simulink model "TORQUECONTROL"  (R2024b)
settings: configuration reference "STM32H7_Config" (kept outside this file)
settings Model: DataDictionary=Master_Dictionary.sldd  EnableAccessToBaseWorkspace=off  Creator=torni  LastModifiedBy=William
settings ConfigSetRef: SourceName=STM32H7_Config

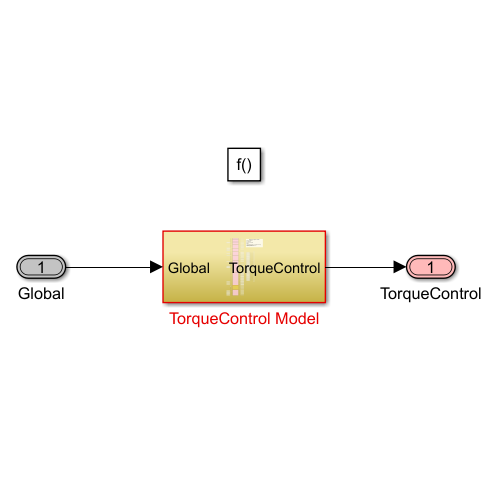
[thumbnail: Simulink's stored preview of the top-level diagram]
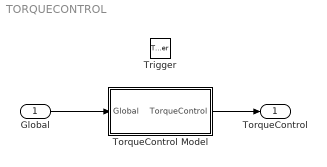
== system TORQUECONTROL ==
  "Global " : Inport  OutDataTypeStr=Bus: Global
  Trigger : TriggerPort  TriggerType=function-call  VariantControl=Variant  PortDimensions=1
  "TorqueControl Model " : Subsystem
  TorqueControl : Outport  OutDataTypeStr=Bus: TorqueControlBus  VectorParamsAs1DForOutWhenUnconnected=off
  wires:
  "Global "/1 -> "TorqueControl Model "/1(Global)
  "TorqueControl Model "/1(TorqueControl) -> TorqueControl/1

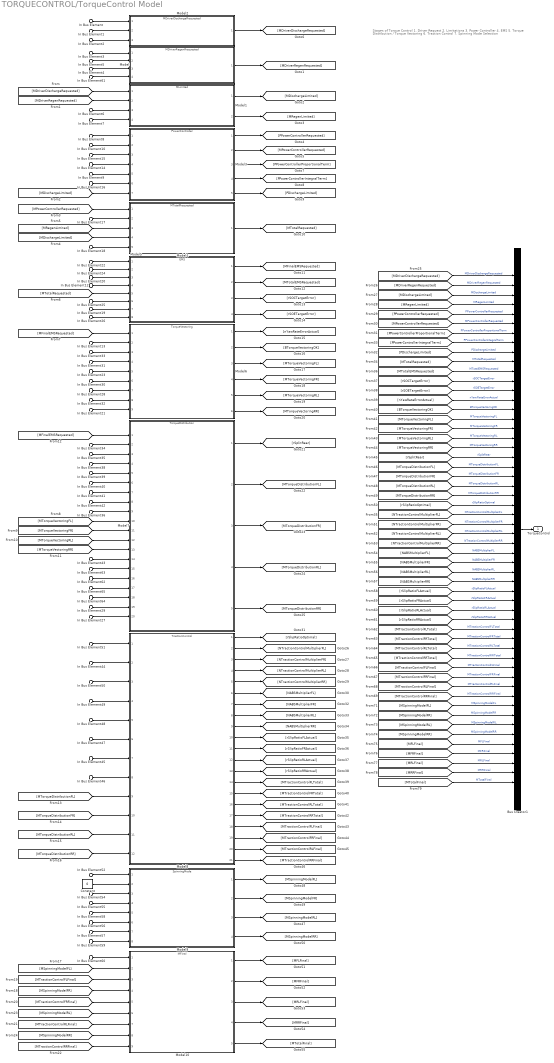
== system TORQUECONTROL/TorqueControl Model  ==
  note: Stages of Torque Control
      | 1. Driver Request
      | 2. Limitations
      | 3. Power Controller
      | 4. EMS
      | 5. Torque Distribution / Torque Vectoring
      | 6. Traction Control
      | 7. Spinning Mode Selection
  In Bus Element{,9,17,28,35,52} (6 alike) : Inport  PortName=Global  Element=SystemsBus.rThrottlePedal
  In Bus Element{1,8,19,23,34,44} (6 alike) : Inport  PortName=Global  Element=SystemsBus.vChassis
  In Bus Element2 : Inport  PortName=Global  Element=SystemsBus.NThrottleMap
  In Bus Element29 : Inport  PortName=Global  Element=SystemsBus.NThrottleMap
  In Bus Element4 : Inport  PortName=Global  Element=SystemsBus.rRegenPaddle
  In Bus Element38 : Inport  PortName=Global  Element=SystemsBus.rRegenPaddle
  In Bus Element5 : Inport  PortName=Global  Element=SystemsBus.PRegen
  In Bus Element10 : Inport  PortName=Global  Element=SystemsBus.NPowerControllerKpSelector
  In Bus Element14 : Inport  PortName=Global  Element=SystemsBus.PActual
  In Bus Element18 : Inport  PortName=Global  Element=SystemsBus.PActual
  In Bus Element16 : Inport  PortName=Global  Element=SystemsBus.PDischarge
  In Bus Element20 : Inport  PortName=Global  Element=SystemsBus.BEMS1000mPoint
  In Bus Element22 : Inport  PortName=Global  Element=SystemsBus.BEMSActivated
  In Bus Element27 : Inport  PortName=Global  Element=SystemsBus.BEMSActivated
  In Bus Element24 : Inport  PortName=Global  Element=SystemsBus.rSOC
  In Bus Element25 : Inport  PortName=Global  Element=SystemsBus.rSOE
  In Bus Element30 : Inport  PortName=Global  Element=SystemsBus.pBrakeMax
  In Bus Element55 : Inport  PortName=Global  Element=SystemsBus.pBrakeMax
  In Bus Element31 : Inport  PortName=Global  Element=SystemsBus.aSteeringAngle
  In Bus Element32 : Inport  PortName=Global  Element=SystemsBus.BTorqueVectoringActivated
  In Bus Element43 : Inport  PortName=Global  Element=SystemsBus.BTorqueVectoringActivated
  In Bus Element33 : Inport  PortName=Global  Element=SystemsBus.rTorqueVectoringMultiplier
  In Bus Element39 : Inport  PortName=Global  Element=SystemsBus.BEncoderErrorRear
  In Bus Element40 : Inport  PortName=Global  Element=SystemsBus.BEncoderErrorFront
  In Bus Element41 : Inport  PortName=Global  Element=SystemsBus.PEngineBraking
  In Bus Element49 : Inport  PortName=Global  Element=SystemsBus.NTractionControlKpSelector
  In Bus Element50 : Inport  PortName=Global  Element=SystemsBus.BTractionControlActivated
  In Bus Element51 : Inport  PortName=Global  Element=SystemsBus.rSteeringAngle
  In Bus Element60 : Inport  PortName=Global  Element=SystemsBus.BSpinningModelActivated
  In Bus Element12 : Inport  PortName=Global  Element=SystemsBus.BEMS995mPoint
  In Bus Element3 : Inport  PortName=Global  Element=BMSSignalsBus.IIVTS
  In Bus Element6 : Inport  PortName=Global  Element=LimitationsBus.rDischargeDerate
  In Bus Element26 : Inport  PortName=Global  Element=LimitationsBus.rDischargeDerate
  In Bus Element7 : Inport  PortName=Global  Element=LimitationsBus.rRegenDerate
  In Bus Element42 : Inport  PortName=Global  Element=LimitationsBus.rRegenDerate
  In Bus Element62 : Inport  PortName=Global  Element=LimitationsBus.rTSTemperatureDerateFR
  In Bus Element63 : Inport  PortName=Global  Element=LimitationsBus.rTSTemperatureDerateFL
  In Bus Element64 : Inport  PortName=Global  Element=LimitationsBus.rTSTemperatureDerateRR
  In Bus Element65 : Inport  PortName=Global  Element=LimitationsBus.rTSTemperatureDerateRL
  In Bus Element15 : Inport  PortName=Global  Element=InverterSignalsBus.InverterRLSignalsBus.VDCInvRL
  In Bus Element36 : Inport  PortName=Global  Element=InverterSignalsBus.InverterRLSignalsBus.VDCInvRL
  In Bus Element61 : Inport  PortName=Global  Element=InverterSignalsBus.InverterRLSignalsBus.VDCInvRL
  In Bus Element58 : Inport  PortName=Global  Element=InverterSignalsBus.InverterRLSignalsBus.nMotorRL
  In Bus Element56 : Inport  PortName=Global  Element=InverterSignalsBus.InverterFLSignalsBus.nMotorFL
  In Bus Element57 : Inport  PortName=Global  Element=InverterSignalsBus.InverterFRSignalsBus.nMotorFR
  In Bus Element59 : Inport  PortName=Global  Element=InverterSignalsBus.InverterRRSignalsBus.nMotorRR
  In Bus Element45 : Inport  PortName=Global  Element=WheelSpeedsBus.vWheelRL
  In Bus Element46 : Inport  PortName=Global  Element=WheelSpeedsBus.vWheelRR
  In Bus Element47 : Inport  PortName=Global  Element=WheelSpeedsBus.vWheelFR
  In Bus Element48 : Inport  PortName=Global  Element=WheelSpeedsBus.vWheelFL
  In Bus Element54 : Inport  PortName=Global  Element=StateflowBus.BReadyToDrive
  In Bus Element13 : Inport  PortName=Global  Element=GPSIMUSignalsBus.gLongitudinalOXTSIMU
  In Bus Element21 : Inport  PortName=Global  Element=GPSIMUSignalsBus.nYawRateOXTSIMU
  Bus Creator1 : BusCreator  Inputs=54  OutDataTypeStr=Bus: TorqueControlBus
  Constant : Constant  Value=0  OutDataTypeStr=boolean
  Model : ModelReference  ModelNameDialog=MDriverRegenRequested.slx  SimulationMode=Normal  ModelReferenceVersion=13.5
  Model1 : ModelReference  ModelNameDialog=MLimited.slx  SimulationMode=Normal  ModelReferenceVersion=13.5
  Model10 : ModelReference  ModelNameDialog=MFinal.slx  SimulationMode=Normal  ModelReferenceVersion=13.5
  Model2 : ModelReference  ModelNameDialog=MDriverDischargeRequested.slx  SimulationMode=Normal  ModelReferenceVersion=13.5
  Model3 : ModelReference  ModelNameDialog=PowerController.slx  SimulationMode=Normal  ModelReferenceVersion=13.5
  Model4 : ModelReference  ModelNameDialog=MTotalRequested.slx  SimulationMode=Normal  ModelReferenceVersion=13.5
  Model5 : ModelReference  ModelNameDialog=EMS.slx  SimulationMode=Normal  ModelReferenceVersion=13.5
  Model6 : ModelReference  ModelNameDialog=TorqueVectoring.slx  SimulationMode=Normal  ModelReferenceVersion=13.5
  Model7 : ModelReference  ModelNameDialog=TorqueDistribution.slx  SimulationMode=Normal  ModelReferenceVersion=13.5
  Model8 : ModelReference  ModelNameDialog=TractionControl.slx  SimulationMode=Normal  ModelReferenceVersion=13.6
  Model9 : ModelReference  ModelNameDialog=SpinningMode.slx  SimulationMode=Normal  ModelReferenceVersion=13.5
  TorqueControl : Outport  OutDataTypeStr=Bus: TorqueControlBus  VectorParamsAs1DForOutWhenUnconnected=off
  wires:
  In Bus Element/1 -> Model2/1
  [MDriverDischargeRequested] -> Model1/1
  Model2/1 -> [MDriverDischargeRequested]
  In Bus Element2/1 -> Model2/3
  In Bus Element1/1 -> Model2/2
  In Bus Element3/1 -> Model/1
  In Bus Element5/1 -> Model/2
  In Bus Element4/1 -> Model/3
  Model/1 -> [MDriverRegenRequested]
  [MDriverRegenRequested] -> Model1/2
  In Bus Element7/1 -> Model1/4
  In Bus Element6/1 -> Model1/3
  Model1/1 -> [MDischargeLimited]
  Model1/2 -> [MRegenLimited]
  Model3/1 -> [PPowerControllerRequested]
  Model3/2 -> [MPowerControllerRequested]
  Model3/3 -> [PPowerControllerProportionalTerm]
  Model3/4 -> [PPowerControllerIntegralTerm]
  Model3/5 -> [PDischargeLimited]
  [MPowerControllerRequested] -> Model4/1
  In Bus Element17/1 -> Model4/2
  In Bus Element18/1 -> Model4/5
  [MDischargeLimited] -> Model4/4
  [MRegenLimited] -> Model4/3
  Model4/1 -> [MTotalRequested]
  In Bus Element12/1 -> Model5/4
  In Bus Element20/1 -> Model5/3
  In Bus Element22/1 -> Model5/1
  [MTotalRequested] -> Model5/5
  In Bus Element25/1 -> Model5/6
  Model5/1 -> [MFinalEMSRequested]
  Model5/2 -> [MTotalEMSRequested]
  Model5/3 -> [rSOCTargetError]
  Model5/4 -> [rSOETargetError]
  In Bus Element13/1 -> Model6/2
  [MFinalEMSRequested] -> Model6/1
  In Bus Element31/1 -> Model6/4
  In Bus Element23/1 -> Model6/5
  In Bus Element30/1 -> Model6/6
  In Bus Element28/1 -> Model6/7
  In Bus Element32/1 -> Model6/8
  In Bus Element21/1 -> Model6/9
  In Bus Element33/1 -> Model6/3
  Model6/1 -> [nYawRateErrorActual]
  Model6/2 -> [BTorqueVectoringOK]
  Model6/3 -> [MTorqueVectoringFL]
  Model6/4 -> [MTorqueVectoringFR]
  Model6/5 -> [MTorqueVectoringRL]
  Model6/6 -> [MTorqueVectoringRR]
  Model7/1 -> [rSplitRear]
  Model7/2 -> [MTorqueDistributionFL]
  Model7/3 -> [MTorqueDistributionFR]
  Model7/4 -> [MTorqueDistributionRL]
  Model7/5 -> [MTorqueDistributionRR]
  Model8/1 -> [rSlipRatioOptimal]
  In Bus Element47/1 -> Model8/6
  In Bus Element56/1 -> Model9/6
  In Bus Element57/1 -> Model9/7
  In Bus Element59/1 -> Model9/8
  In Bus Element58/1 -> Model9/5
  In Bus Element52/1 -> Model9/1
  Constant/1 -> Model9/2
  In Bus Element55/1 -> Model9/4
  Model9/1 -> [MSpinningModelFL]
  Model9/2 -> [MSpinningModelFR]
  Model9/3 -> [MSpinningModelRL]
  Model9/4 -> [MSpinningModelRR]
  Model10/1 -> [MFLFinal]
  Model10/2 -> [MFRFinal]
  Model10/3 -> [MRLFinal]
  Model10/4 -> [MRRFinal]
  [MSpinningModelFL] -> Model10/2
  [MSpinningModelFR] -> Model10/4
  In Bus Element60/1 -> Model10/1
  [MTractionControlFLFinal] -> Model10/3
  [MTractionControlFRFinal] -> Model10/5
  [MTractionControlRLFinal] -> Model10/7
  [MTractionControlRRFinal] -> Model10/9
  [MSpinningModelRL] -> Model10/6
  [MSpinningModelRR] -> Model10/8
  Bus Creator1/1 -> TorqueControl/1
  [MDriverDischargeRequested] -> Bus Creator1/1  "MDriverDischargeRequested"
  [MDriverRegenRequested] -> Bus Creator1/2  "MDriverRegenRequested"
  [MDischargeLimited] -> Bus Creator1/3  "MDischargeLimited"
  [MRegenLimited] -> Bus Creator1/4  "MRegenLimited"
  [PPowerControllerRequested] -> Bus Creator1/5  "PPowerControllerRequested"
  [MPowerControllerRequested] -> Bus Creator1/6  "MPowerControllerRequested"
  [PPowerControllerProportionalTerm] -> Bus Creator1/7  "PPowerControllerProportionalTerm"
  [PPowerControllerIntegralTerm] -> Bus Creator1/8  "PPowerControllerIntegralTerm"
  [PDischargeLimited] -> Bus Creator1/9  "PDischargeLimited"
  [MTotalRequested] -> Bus Creator1/10  "MTotalRequested"
  [MTotalEMSRequested] -> Bus Creator1/11  "MTotalEMSRequested"
  [rSOCTargetError] -> Bus Creator1/12  "rSOCTargetError"
  [rSOETargetError] -> Bus Creator1/13  "rSOETargetError"
  [nYawRateErrorActual] -> Bus Creator1/14  "nYawRateErrorActual"
  [BTorqueVectoringOK] -> Bus Creator1/15  "BTorqueVectoringOK"
  [MTorqueVectoringFL] -> Bus Creator1/16  "MTorqueVectoringFL"
  [MTorqueVectoringFR] -> Bus Creator1/17  "MTorqueVectoringFR"
  [MTorqueVectoringRL] -> Bus Creator1/18  "MTorqueVectoringRL"
  [MTorqueVectoringRR] -> Bus Creator1/19  "MTorqueVectoringRR"
  [rSplitRear] -> Bus Creator1/20  "rSplitRear"
  [MTorqueDistributionFL] -> Bus Creator1/21  "MTorqueDistributionFL"
  [MTorqueDistributionFR] -> Bus Creator1/22  "MTorqueDistributionFR"
  [MTorqueDistributionRL] -> Bus Creator1/23  "MTorqueDistributionRL"
  [MTorqueDistributionRR] -> Bus Creator1/24  "MTorqueDistributionRR"
  [rSlipRatioOptimal] -> Bus Creator1/25  "rSlipRatioOptimal"
  [MSpinningModelFL] -> Bus Creator1/46  "MSpinningModelFL"
  [MSpinningModelFR] -> Bus Creator1/47  "MSpinningModelFR"
  [MSpinningModelRL] -> Bus Creator1/48  "MSpinningModelRL"
  [MSpinningModelRR] -> Bus Creator1/49  "MSpinningModelRR"
  [MFLFinal] -> Bus Creator1/50  "MFLFinal"
  [MFRFinal] -> Bus Creator1/51  "MFRFinal"
  [MRLFinal] -> Bus Creator1/52  "MRLFinal"
  [MRRFinal] -> Bus Creator1/53  "MRRFinal"
  Model10/5 -> [MTotalFinal]
  [MTotalFinal] -> Bus Creator1/54  "MTotalFinal"
  In Bus Element19/1 -> Model5/7
  In Bus Element54/1 -> Model9/3
  In Bus Element24/1 -> Model5/2
  In Bus Element61/1 -> Model/4
  In Bus Element8/1 -> Model3/1
  In Bus Element10/1 -> Model3/2
  In Bus Element15/1 -> Model3/3
  [MDischargeLimited] -> Model3/7
  In Bus Element26/1 -> Model5/8
  In Bus Element14/1 -> Model3/4
  In Bus Element9/1 -> Model3/5
  In Bus Element16/1 -> Model3/6
  In Bus Element48/1 -> Model8/5
  In Bus Element44/1 -> Model8/2
  In Bus Element49/1 -> Model8/4
  In Bus Element50/1 -> Model8/3
  In Bus Element45/1 -> Model8/7
  In Bus Element46/1 -> Model8/8
  In Bus Element51/1 -> Model8/1
  [MTorqueDistributionRR] -> Model8/12
  [MTorqueDistributionRL] -> Model8/11
  [MTorqueDistributionFR] -> Model8/10
  [MTorqueDistributionFL] -> Model8/9
  Model8/2 -> [NTractionControlMultiplierFL]
  Model8/5 -> [NTractionControlMultiplierRR]
  Model8/4 -> [NTractionControlMultiplierRL]
  Model8/3 -> [NTractionControlMultiplierFR]
  Model8/6 -> [NABSMultiplierFL]
  Model8/7 -> [NABSMultiplierFR]
  Model8/8 -> [NABSMultiplierRL]
  Model8/9 -> [NABSMultiplierRR]
  Model8/10 -> [rSlipRatioFLActual]
  Model8/11 -> [rSlipRatioFRActual]
  Model8/12 -> [rSlipRatioRLActual]
  Model8/13 -> [rSlipRatioRRActual]
  Model8/14 -> [MTractionControlFLTotal]
  Model8/15 -> [MTractionControlFRTotal]
  Model8/16 -> [MTractionControlRLTotal]
  Model8/17 -> [MTractionControlRRTotal]
  Model8/18 -> [MTractionControlFLFinal]
  Model8/19 -> [MTractionControlFRFinal]
  Model8/20 -> [MTractionControlRLFinal]
  Model8/21 -> [MTractionControlRRFinal]
  [NTractionControlMultiplierFL] -> Bus Creator1/26  "NTractionControlMultiplierFL"
  [NTractionControlMultiplierFR] -> Bus Creator1/27  "NTractionControlMultiplierFR"
  [NTractionControlMultiplierRL] -> Bus Creator1/28  "NTractionControlMultiplierRL"
  [NTractionControlMultiplierRR] -> Bus Creator1/29  "NTractionControlMultiplierRR"
  [NABSMultiplierFL] -> Bus Creator1/30  "NABSMultiplierFL"
  [NABSMultiplierFR] -> Bus Creator1/31  "NABSMultiplierFR"
  [NABSMultiplierRL] -> Bus Creator1/32  "NABSMultiplierRL"
  [NABSMultiplierRR] -> Bus Creator1/33  "NABSMultiplierRR"
  [rSlipRatioFLActual] -> Bus Creator1/34  "rSlipRatioFLActual"
  [rSlipRatioFRActual] -> Bus Creator1/35  "rSlipRatioFRActual"
  [rSlipRatioRLActual] -> Bus Creator1/36  "rSlipRatioRLActual"
  [rSlipRatioRRActual] -> Bus Creator1/37  "rSlipRatioRRActual"
  [MTractionControlFLTotal] -> Bus Creator1/38  "MTractionControlFLTotal"
  [MTractionControlFRTotal] -> Bus Creator1/39  "MTractionControlFRTotal"
  [MTractionControlRLTotal] -> Bus Creator1/40  "MTractionControlRLTotal"
  [MTractionControlRRTotal] -> Bus Creator1/41  "MTractionControlRRTotal"
  In Bus Element29/1 -> Model7/19
  [MTractionControlFLFinal] -> Bus Creator1/42  "MTractionControlFLFinal"
  [MTractionControlFRFinal] -> Bus Creator1/43  "MTractionControlFRFinal"
  [MTractionControlRLFinal] -> Bus Creator1/44  "MTractionControlRLFinal"
  [MTractionControlRRFinal] -> Bus Creator1/45  "MTractionControlRRFinal"
  In Bus Element35/1 -> Model7/3
  In Bus Element38/1 -> Model7/4
  In Bus Element39/1 -> Model7/5
  In Bus Element40/1 -> Model7/6
  In Bus Element41/1 -> Model7/7
  In Bus Element42/1 -> Model7/8
  In Bus Element36/1 -> Model7/9
  [MTorqueVectoringFL] -> Model7/10
  [MTorqueVectoringFR] -> Model7/11
  [MTorqueVectoringRL] -> Model7/12
  [MTorqueVectoringRR] -> Model7/13
  In Bus Element43/1 -> Model7/14
  In Bus Element64/1 -> Model7/18
  In Bus Element65/1 -> Model7/17
  In Bus Element62/1 -> Model7/16
  In Bus Element63/1 -> Model7/15
  In Bus Element27/1 -> Model7/20
  In Bus Element34/1 -> Model7/2
  [MFinalEMSRequested] -> Model7/1
